simulink model "buck_closed_loop_discrete"  (Simulink 4.0)
settings: Solver=ode45  StartTime=0  StopTime=0.003  MaxStep=0.1e-6  RelTol=1e-3
libraries: simulink x1
settings Model: LastModifiedBy=Dragan Maksimovic  BooleanDataType=on

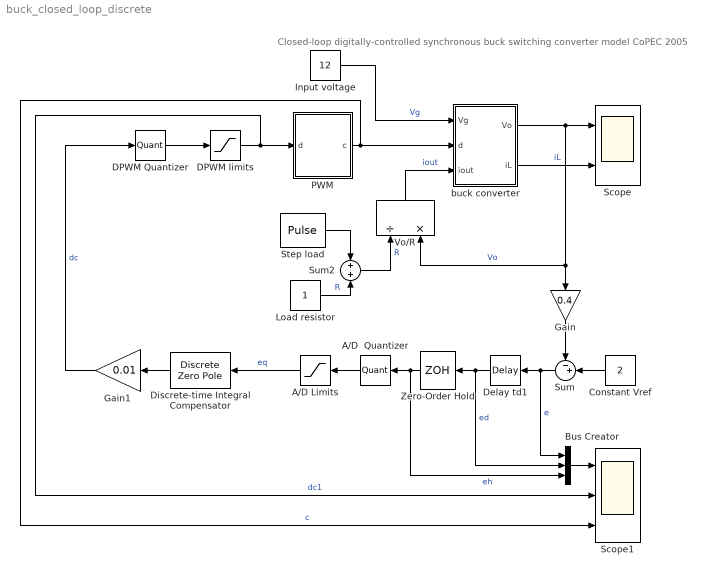
== system buck_closed_loop_discrete ==
  note: Closed-loop digitally-controlled synchronous buck switching converter model
      | CoPEC 2005
  A/D Limits : Saturate  Orientation=left  UpperLimit=1  LowerLimit=-1  LinearizeAsGain=on
  A/D  Quantizer : Quantizer  Orientation=left  QuantizationInterval=1/64  LinearizeAsGain=on
  Bus Creator : BusCreator  Inputs=3
  Constant Vref : Constant  Orientation=left  Value=2
  DPWM Quantizer : Quantizer  QuantizationInterval=1/1024  LinearizeAsGain=on
  DPWM limits : Saturate  UpperLimit=0.8  LowerLimit=0.0  LinearizeAsGain=on
  Delay td1 : TransportDelay  Orientation=left  DelayTime=4e-6  InitialInput=0  BufferSize=1024  PadeOrder=0
  Discrete-time Integral Compensator : DiscreteZeroPole  Orientation=left  Zeros=[0]  Poles=[1]  Gain=1  SampleTime=-1
  Gain : Gain  Orientation=down  Gain=0.4  Multiplication=Element-wise(K.*u)  SaturateOnIntegerOverflow=on
  Gain1 : Gain  Orientation=left  Gain=0.01  Multiplication=Element-wise(K.*u)  SaturateOnIntegerOverflow=on
  Input voltage : Constant  Value=12
  Load resistor : Constant  Value=1
  PWM : Subsystem  SimViewingDevice=off
      settings: Permissions=ReadWrite  RTWFcnNameOpts=Auto  RTWFileNameOpts=Auto
  Scope : Scope  NumInputPorts=2
      settings: TimeRange=0.003  YMin=4.5~-5  YMax=5.5~15  SaveToWorkspace=off  SaveName=ScopeData  MaxDataPoints=5000
  Scope1 : Scope  NumInputPorts=3
      settings: TimeRange=4.99810664347834e-005  YMin=0~0.428~-0.5  YMax=0.1~0.432~1.5  SaveToWorkspace=off  SaveName=ScopeData2  MaxDataPoints=5000
  Step load : DiscretePulseGenerator  PulseType=Time-based  Amplitude=1  Period=0.002  PulseWidth=50  PhaseDelay=0  SampleTime=1
  Sum : Sum  Orientation=left  Inputs=-+|  SaturateOnIntegerOverflow=on
  Sum2 : Sum  Inputs=+|+  SaturateOnIntegerOverflow=on
  Vo/R : Product  Orientation=up  Inputs=/*  Multiplication=Element-wise(.*)  SaturateOnIntegerOverflow=on
  Zero-Order Hold : ZeroOrderHold  Orientation=left  SampleTime=1e-5
  buck converter : Subsystem  SimViewingDevice=off
      settings: Permissions=ReadWrite  RTWFcnNameOpts=Auto  RTWFileNameOpts=Auto
  wires:
  Input voltage/1 -> buck converter/1(Vg)  "Vg"
  buck converter/1(Vo) -> Scope/1, Vo/R/2, Gain/1  "Vo"
  buck converter/2(iL) -> Scope/2  "iL"
  PWM/1(c) -> buck converter/2(d), Scope1/3  "c"
  Vo/R/1 -> buck converter/3(iout)  "iout"
  Gain/1 -> Sum/1
  Constant Vref/1 -> Sum/2
  Step load/1 -> Sum2/1
  Load resistor/1 -> Sum2/2  "R"
  Sum2/1 -> Vo/R/1  "R"
  DPWM Quantizer/1 -> DPWM limits/1
  DPWM limits/1 -> PWM/1(d), Scope1/2  "dc1"
  A/D Limits/1 -> Discrete-time Integral Compensator/1  "eq"
  A/D  Quantizer/1 -> A/D Limits/1
  Zero-Order Hold/1 -> A/D  Quantizer/1, Bus Creator/3  "eh"
  Delay td1/1 -> Zero-Order Hold/1, Bus Creator/2  "ed"
  Sum/1 -> Delay td1/1, Bus Creator/1  "e"
  Bus Creator/1 -> Scope1/1
  Gain1/1 -> DPWM Quantizer/1  "dc"
  Discrete-time Integral Compensator/1 -> Gain1/1

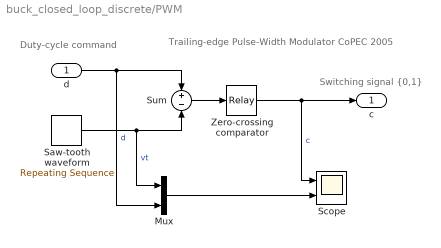
== system buck_closed_loop_discrete/PWM ==
  note: Duty-cycle
      | command
  note: Switching signal {0,1}
  note: Trailing-edge Pulse-Width Modulator
      | CoPEC 2005
  d : Inport  Port=1  PortDimensions=-1  SampleTime=-1  DataType=auto
      settings: SignalType=auto
  Mux : Mux  Inputs=2
  Saw-tooth waveform : simulink/Sources/Repeating Sequence  rep_seq_t=[0 0.001e-5 1e-5]  rep_seq_y=[1 0 1]
  Scope : Scope  NumInputPorts=2
      settings: TimeRange=auto  YMin=0~0  YMax=1.5~1.5  SaveToWorkspace=off  MaxDataPoints=5000
  Sum : Sum  Inputs=+|-  SaturateOnIntegerOverflow=on
  Zero-crossing comparator : Relay  OnSwitchValue=eps  OffSwitchValue=eps  OnOutputValue=1  OffOutputValue=0
  c : Outport  Port=1
  wires:
  Saw-tooth waveform/1 -> Mux/1, Sum/2  "vt"
  d/1 -> Mux/2, Sum/1  "d"
  Zero-crossing comparator/1 -> c/1, Scope/1  "c"
  Sum/1 -> Zero-crossing comparator/1
  Mux/1 -> Scope/2

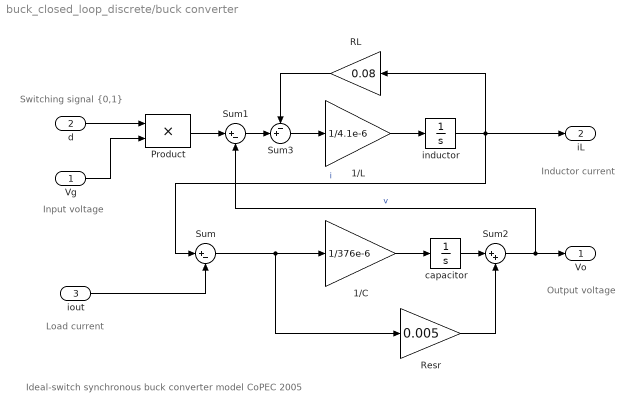
== system buck_closed_loop_discrete/buck converter ==
  note: Load current
  note: Input voltage
  note: Inductor current
  note: Output voltage
  note: Switching signal {0,1}
  note: Ideal-switch synchronous buck converter model
      | CoPEC 2005
  Vg : Inport  Port=1  PortDimensions=-1  SampleTime=-1  DataType=auto
      settings: SignalType=auto
  d : Inport  Port=2  PortDimensions=-1  SampleTime=-1  DataType=auto
      settings: SignalType=auto
  iout : Inport  Port=3  PortDimensions=-1  SampleTime=-1  DataType=auto
      settings: SignalType=auto
  1/C : Gain  Gain=1/376e-6  Multiplication=Element-wise(K.*u)  SaturateOnIntegerOverflow=on
  1/L : Gain  Gain=1/4.1e-6  Multiplication=Element-wise(K.*u)  SaturateOnIntegerOverflow=on
  Product : Product  Inputs=2  Multiplication=Element-wise(.*)  SaturateOnIntegerOverflow=on
  RL : Gain  Orientation=left  Gain=0.08  Multiplication=Element-wise(K.*u)  SaturateOnIntegerOverflow=on
  Resr : Gain  Gain=0.005  Multiplication=Element-wise(K.*u)  SaturateOnIntegerOverflow=on
  Sum : Sum  Inputs=|+-  SaturateOnIntegerOverflow=on
  Sum1 : Sum  Inputs=|+-  SaturateOnIntegerOverflow=on
  Sum2 : Sum  Inputs=|++  SaturateOnIntegerOverflow=on
  Sum3 : Sum  Inputs=-+|  SaturateOnIntegerOverflow=on
  capacitor : Integrator  ExternalReset=none  InitialConditionSource=internal  InitialCondition=0  LimitOutput=off  UpperSaturationLimit=inf  LowerSaturationLimit=-inf  ShowSaturationPort=off  ShowStatePort=off  AbsoluteTolerance=auto
  inductor : Integrator  ExternalReset=none  InitialConditionSource=internal  InitialCondition=0  LimitOutput=off  UpperSaturationLimit=inf  LowerSaturationLimit=-inf  ShowSaturationPort=off  ShowStatePort=off  AbsoluteTolerance=auto
  Vo : Outport  Port=1
  iL : Outport  Port=2
  wires:
  iout/1 -> Sum/2
  d/1 -> Product/1
  Resr/1 -> Sum2/2
  capacitor/1 -> Sum2/1
  Sum3/1 -> 1/L/1
  RL/1 -> Sum3/1
  Sum1/1 -> Sum3/2
  Sum2/1 -> Sum1/2, Vo/1  "v"
  Product/1 -> Sum1/1
  inductor/1 -> Sum/1, RL/1, iL/1  "i"
  1/L/1 -> inductor/1
  Sum/1 -> 1/C/1, Resr/1
  1/C/1 -> capacitor/1
  Vg/1 -> Product/2
